simulink model "Final_EWASP_VC"  (R2022a)
settings: Solver=ode1  StartTime=0.0  StopTime=24*3600  FixedStep=10  RelTol=1e-3
values from neighbouring files (symbols this model uses):
  Aux_Threshold = 52    [Setup_Code_EWASP_VC.m]
  buildingAge = 2005    [Setup_Code_EWASP_VC.m]
  ceilingHeight = 2.4    [Setup_Code_EWASP_VC.m]
  conductiveHconnectMatrix = [ ... (first row only)    [Setup_Code_EWASP_VC.m]
  cRoofGreen = 100000    [Setup_Code_EWASP_VC.m]
  Defrost_After_Time = 30    [Setup_Code_EWASP_VC.m]
  DHWDemandProfile = occFreegainHotwaterElecTestPassiveOcc3(:,3)    [Setup_Code_EWASP_VC.m]
  Elec_Max = Elec_Max*(30/24.2)    [Setup_Code_EWASP_VC.m]
  Elec_Mid = Elec_Mid*(30/24.2)    [Setup_Code_EWASP_VC.m]
  Elec_Min = Elec_Min*(30/24.2)    [Setup_Code_EWASP_VC.m]
  ElecDemandProfile = occFreegainHotwaterElecTestPassiveOcc3(:,4)    [Setup_Code_EWASP_VC.m]
  ElecFixed = [Elec_Max(6,2) Elec_Max(6,4) Elec_Max(6,6) Elec_Max(6,7) ... (first row only)    [Setup_Code_EWASP_VC.m]
  floorOrCeilingArea = floorOrCeilingArea*1.15    [Setup_Code_EWASP_VC.m]
  forceCold = 0    [Setup_Code_EWASP_VC.m]
  freegain = occFreegainHotwaterElecTestPassiveOcc3(:,2)-max(occupancy)*25    [Setup_Code_EWASP_VC.m]
  furnitureModelOn = 1    [Setup_Code_EWASP_VC.m]
  Heat_Max = Heat_Max*(30/24.2)    [Setup_Code_EWASP_VC.m]
  Heat_Mid = Heat_Mid*(30/24.2)    [Setup_Code_EWASP_VC.m]
  Heat_Min = Heat_Min*(30/24.2)    [Setup_Code_EWASP_VC.m]
  HeatFixed = [Heat_Max(6,2) Heat_Max(6,4) Heat_Max(6,6) Heat_Max(6,7) ... (first row only)    [Setup_Code_EWASP_VC.m]
  HeatingOnProfile = repmat(HeatingOnProfile,365,1)    [Setup_Code_EWASP_VC.m]
  HEX_ReturnLowerLimit = 52.5    [Setup_Code_EWASP_VC.m]
  HEX_ReturnUpperLimit = 55    [Setup_Code_EWASP_VC.m]
  LeakMultiplier = 1+(2*(rand()-0.5)/10)    [Setup_Code_EWASP_VC.m]
  loopCap = 15    [Setup_Code_EWASP_VC.m]
  maxOcc = max(occupancyProfile)    [Setup_Code_EWASP_VC.m]
  NESW_wallArea = max(NESW_Lengths*ceilingHeight-NESW_Windows,0)    [Setup_Code_EWASP_VC.m]
  NESW_Windows = [ ... (first row only)    [Setup_Code_EWASP_VC.m]
  numRooms = roomCount    [Setup_Code_EWASP_VC.m]
  offsetDays = 0    [Setup_Code_EWASP_VC.m]
  pumpChoice = pumpChoices(MinIndex,1)    [Setup_Code_EWASP_VC.m]
  pumpRamp = 180    [Setup_Code_EWASP_VC.m]
  ReturnLowerLimit = 37.5    [Setup_Code_EWASP_VC.m]
  ReturnUpperLimit = 40    [Setup_Code_EWASP_VC.m]
  RoofIrradiance = Flat_NS_EW_RoofIrradiance(:,1)    [Setup_Code_EWASP_VC.m]
  roofStartTemp = ones(11,1)*20    [Setup_Code_EWASP_VC.m]
  rooftype = 0    [Setup_Code_EWASP_VC.m]
  RoomDataMatrix = [zeros(1,12);ones(1,12)*wallDensity;zeros(1,12);ones(1,12)*wallU;ones(1,12)*windowU;ones(1,12)*floorU;ones(1,12)*ceilingU;zeros(1,12);windowArea, 0;floorOrCeilingArea;zeros(1,12);floorOrCeilingArea*ceilingHeight]    [Setup_Code_EWASP_VC.m]
  roomVol = roomVol*1.15    [Setup_Code_EWASP_VC.m]
  slabStartTemp = (GroundTempTimeSeries(offsetDays*1440+1,1)+thermostatSetting)/2    [Setup_Code_EWASP_VC.m]
  SlackRequest = zeros(1440,1)    [Setup_Code_EWASP_VC.m]
  SolarThermalExists = 0    [Setup_Code_EWASP_VC.m]
  SourceFixed = HeatFixed-ElecFixed    [Setup_Code_EWASP_VC.m]
  StateSeries = StateSeriesGenerator(22,7,1)    [Setup_Code_EWASP_VC.m]
  Tank_Lower_Temp = 49.5    [Setup_Code_EWASP_VC.m]
  Tank_Upper_Temp = 52    [Setup_Code_EWASP_VC.m]
  Tank_Volume_m3 = 0.15    [Setup_Code_EWASP_VC.m]
  TankHeatHour = randi([1 5])-1    [Setup_Code_EWASP_VC.m]
  thermostatSetting = 20.0    (= 20)    [Setup_Code_EWASP_VC.m]
  upDown = [0;0;0;0;1;1;1;1;1;1;1]    [Setup_Code_EWASP_VC.m]
  variableASHP = 1    [Setup_Code_EWASP_VC.m]
  wallStartTempExt = thermostatSetting*(0.266+0.00215*outdoorStartTemp+0.018*wallU+0.00113*outdoorStartTemp*wallU+0.0068*wallU^2)    [Setup_Code_EWASP_VC.m]
undefined symbols (not defined in the file or in its folder): a, ceilingU, condUDMatrix, convUDMatrix, deltaPEXPANDED_E, deltaPEXPANDED_E2, deltaPEXPANDED_N, deltaPEXPANDED_N2, deltaPEXPANDED_S, deltaPEXPANDED_S2, deltaPEXPANDED_W, deltaPEXPANDED_W2, DesiredDHWTemp, DesiredFlowTempVsInOutDeltaTemp, DiffuseHorizontal, DiscIntNeverNeededParam, DNI, dwnAndConcrete, DWORK_A_HX, DWORK_CHK_FLU, DWORK_CP_NODE, DWORK_DH, DWORK_FLUID, DWORK_HCON, DWORK_LOSS, DWORK_MDOTDOWN, DWORK_MDOTIN, DWORK_MDOTUP, DWORK_MIX, DWORK_PRESS, DWORK_QDOTIN, DWORK_RHO_NODE, DWORK_TIN, DWORK_TS_OLD, DWORK_V_NODE, GroundTempTimeSeries, HCM, HCM2, HCM_closed, HCM_closed2, intermediateU, IsTop, massFlowMatrix, neighbourMatrix, numericalRoomUse, RadiatorMatrix, room2roomflowmatrix_E, room2roomflowmatrix_E2, room2roomflowmatrix_N, room2roomflowmatrix_N2, room2roomflowmatrix_S, room2roomflowmatrix_S2, room2roomflowmatrix_W, room2roomflowmatrix_W2, StateAirInEXPANDED_E, StateAirInEXPANDED_E2, StateAirInEXPANDED_N, StateAirInEXPANDED_N2, StateAirInEXPANDED_S, StateAirInEXPANDED_S2 ... (+23)
libraries: simulink x6, dspsigops x4, dspmtrx3 x4, carnot x3, spsEdgeDetectorLib x2, dspstat3 x2, powerlib_meascontrol x1, simulink_extras x1
(part 1 of 27)
settings Model: Creator=cpp14rcj  LastModifiedBy=cpp14rcj
settings SolverCC: AlgebraicLoopSolver=TrustRegion  AutoInsertRateTranBlk=on
settings DataIOCC: SaveFormat=Array  ReturnWorkspaceOutputs=off
settings OptimizationCC: DefaultParameterBehavior=Inlined
settings DebuggingCC: UnconnectedInputMsg=warning  UnconnectedOutputMsg=warning  UnconnectedLineMsg=warning  SFMachineParentedDataDiag=warning  ArithmeticOperatorsInVariantConditions=warning
settings SFSimCC: CustomCodeUndefinedFunction=UseInterfaceOnly
settings ConfigComp: PSAutoStubLUT=on

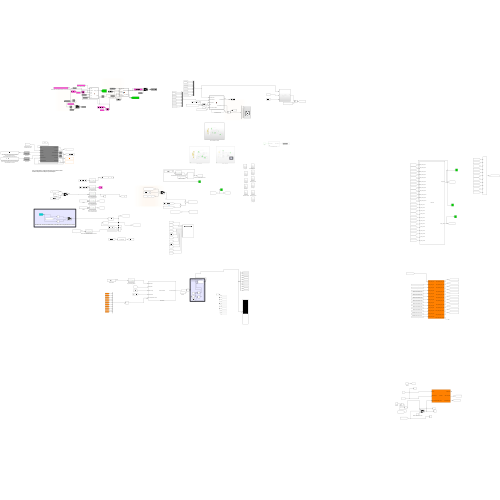
[thumbnail: Simulink's stored preview of the top-level diagram]
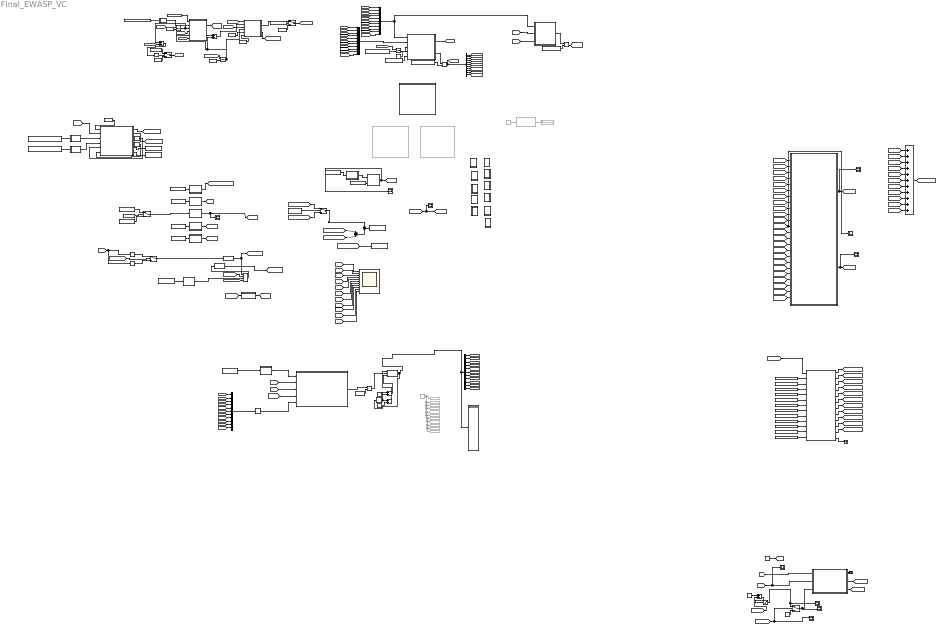
== system Final_EWASP_VC ==
  note: Prevents airflow from altering
      | extremely rapidly
  note: Handles the room thermostat band, and relaxes it if a request to do so is sent
  note: Grey Components: Components that are part of the model
      | White Components: Example Inputs/Outputs
  1 m : Relay  OnSwitchValue=18.1  OffSwitchValue=18  OnOutputValue=0  OffOutputValue=1  OutDataTypeStr=boolean
  1 m10 : Relay  OnSwitchValue=7  OffSwitchValue=1  OutDataTypeStr=boolean
  ASHP_Subsystem : Subsystem  Commented=on
  ASHP_Subsystem_Variable : Subsystem
  Add : Sum  Inputs=11
  Add2 : Sum
  Add3 : Sum  Inputs=+-
  Airflow Model : Subsystem
      mask Display:
      | disp('Air Flow Heat Loss')
      | port_label('input',1,'State Switch')
      | port_label('input',2,'Wind Speed')
      | port_label('input',3,'Outdoor Temp')
      | port_label('input',4,'Wind Direction')
      | port_label('input',5,'Room Temperature Vector')
      | port_label('output',1,'Room Loss Vector')
  CondLossIntermediate : Subsystem  Commented=on
      mask Display:
      | port_label('input',1, 'RoomNum')
      | port_label('output',1,'IntCondGain')
  Constant1 : Constant  Commented=on  Value=0
  Constant10 : Constant  Value=50
  Constant11 : Constant  Value=maxOcc*0.054/2
  Constant12 : Constant  Value=variableASHP
  Constant14 : Constant  Value=0
  Constant2 : Constant  Value=25
  Constant3 : Constant  Value=2.1
  Constant4 : Constant  Commented=on  Value=11
  Constant5 : Constant  Value=25
  Constant6 : Constant  Value=20*ones(11,11)
  Constant7 : Constant  Value=conductiveHconnectMatrix
  Constant8 : Constant  Value=0
  Constant9 : Constant  Value=20
  Data Type Conversion : DataTypeConversion  OutDataTypeStr=double  SaturateOnIntegerOverflow=off  RndMeth=Floor
  Data Type Conversion2 : DataTypeConversion  OutDataTypeStr=double  SaturateOnIntegerOverflow=off  RndMeth=Floor
  Delay3 : Delay  DelayLength=1  InitialCondition=0
  Delay4 : Delay  DelayLength=1  InitialCondition=0
  Delay5 : Delay  DelayLength=1  InitialCondition=0
  Demux : Demux  Outputs=11
  Demux1 : Demux  Outputs=11
  Digital Clock3 : DigitalClock  SampleTime=10
  Discrete-Time Integrator : DiscreteIntegrator  InitialConditionSource=external  InitialCondition=20  SampleTime=-1  ICPrevOutput=DiscIntNeverNeededParam  ICPrevScaledInput=DiscIntNeverNeededParam
  Discrete-Time Integrator1 : DiscreteIntegrator  InitialConditionSource=external  SampleTime=-1  ICPrevOutput=DiscIntNeverNeededParam  ICPrevScaledInput=DiscIntNeverNeededParam
  Display : Display
  Display3 : Display  Commented=on
  GSHP_Subsystem : Subsystem  Commented=on
  Goto11 : Goto  Commented=on  GotoTag=AirLoss5  TagVisibility=global
  Goto12 : Goto  Commented=on  GotoTag=AirLoss6  TagVisibility=global
  Goto16 : Goto  Commented=on  GotoTag=AirLoss7  TagVisibility=global
  Goto18 : Goto  Commented=on  GotoTag=AirLoss8  TagVisibility=global
  Goto19 : Goto  Commented=on  GotoTag=AirLoss9  TagVisibility=global
  Goto20 : Goto  Commented=on  GotoTag=AirLoss10  TagVisibility=global
  Goto21 : Goto  Commented=on  GotoTag=AirLoss11  TagVisibility=global
  Goto5 : Goto  Commented=on  GotoTag=AirLoss1  TagVisibility=global
  Goto7 : Goto  Commented=on  GotoTag=AirLoss2  TagVisibility=global
  Goto8 : Goto  Commented=on  GotoTag=AirLoss3  TagVisibility=global
  Goto9 : Goto  Commented=on  GotoTag=AirLoss4  TagVisibility=global
  Heat sys act?1 : Constant  Value=HeatingOnProfile
  Heat sys act?2 : Constant  Value=StateSeries
  Logical Operator5 : Logic  Inputs=4  AllPortsSameDT=off  OutDataTypeStr=boolean
  MATLAB Function : MATLAB Function  TreatAsAtomicUnit=on
  MATLAB Function1 : MATLAB Function  TreatAsAtomicUnit=on
  MATLAB Function2 : MATLAB Function  TreatAsAtomicUnit=on
  MATLAB Function3 : MATLAB Function  TreatAsAtomicUnit=on
  Massflow when system is off3 : Constant  Value=0
  Massflow when system is on1 : Constant  Value=massFlowMatrix(1,3)
  Massflow when system is on10 : Constant  Value=massFlowMatrix(1,11)
  Massflow when system is on11 : Constant  Value=massFlowMatrix(1,10)
  Massflow when system is on13 : Constant  Value=massFlowMatrix(1,2)
  Massflow when system is on2 : Constant  Value=massFlowMatrix(1,1)
  Massflow when system is on3 : Constant  Value=massFlowMatrix(1,6)
  Massflow when system is on4 : Constant  Value=massFlowMatrix(1,5)
  Massflow when system is on5 : Constant  Value=massFlowMatrix(1,9)
  Massflow when system is on6 : Constant  Value=massFlowMatrix(1,8)
  Massflow when system is on7 : Constant  Value=massFlowMatrix(1,4)
  Massflow when system is on8 : Constant  Value=massFlowMatrix(1,7)
  Massflow when system is on9 : Constant  Value=massFlowMatrix(1,12)
  Minus : Sum  Inputs=+-
  Mux : Mux  Inputs=11
  Mux1 : Mux  Inputs=11
  Offset Independent time series element selector : Subsystem
  Offset Independent time series element selector1 : Subsystem
  Offset Independent time series element selector2 : Subsystem
  Plus : Sum  Inputs=+-
  Plus1 : Sum  Inputs=+-
  Product : Product  Inputs=*/
  Product2 : Product
  Product3 : Product  Inputs=*/
  Product4 : Product  Inputs=*/
  Radiator w/Thermostatic Control : Subsystem  mask{DeltaT_Nominal=40, Power_Nominal=100, TRV_Therm_Setpoint=1000, Water_Volume=10}
      mask prompts: DeltaT_Nominal "DeltaT_Nominal (oC)"; Power_Nominal "Power_Nominal (W)"; TRV_Therm_Setpoint "TRV/Thermostat Setpoint (oC)"; Water_Volume "Water Volume (l)"
      mask Display:
      | disp('Radiator')
      | port_label('input', 1, 'Troom')
      | port_label('input', 2, 'Water Temp In')
      | port_label('input', 3, 'Water Mass Flow Rate (open)')
      | port_label('output', 1, 'Qdot2room')
      | port_label('output', 2, 'Water Temp Out')
      | port_label('output', 3, 'Actual Mass Flow')
      | %image('C:\Users\cpp14rcj\Desktop\MODEL IMAGES\radiator-67-778961.png')
  Relay1 : Relay  OnSwitchValue=thermostatSetting  OffSwitchValue=thermostatSetting-thermostatBand  OnOutputValue=0  OffOutputValue=1  OutDataTypeStr=boolean
  Saturation Dynamic : simulink/Discontinuities/Saturation Dynamic  OutMin=[]  OutMax=[]  OutDataTypeStr=Inherit: Same as second input  OutDataType=fixdt(1, 16)  OutScaling=2^-10  DoSatur=off
  Saturation1 : Saturate  UpperLimit=1000  LowerLimit=0
  Scope{,3,6,10,12..13,16,19} (8 alike) : Scope
  Scope5 : Scope  NumInputPorts=11
  Scope7 : Scope  NumInputPorts=2
  Scope9 : Scope  NumInputPorts=2
  Select Correct Element from Array1 : Subsystem
  Select Correct Element from Array2 : Subsystem
  "Select correct element from array, considering offset" : Subsystem
  "Select correct element from array, considering offset1" : Subsystem
  "Select correct element from array, considering offset2" : Subsystem
  "Select correct element from array, considering offset3" : Subsystem
  "Select correct element from array, considering offset4" : Subsystem
  Selector2 : Selector  NumberOfDimensions=2  InputPortWidth=3  IndexOptions=Index vector (dialog),Index vector (dialog)  Indices=1:11,1  OutputSizes=1,1
  Subsystem : Subsystem
      mask Display:
      | disp('Flow mixer')
      | port_label('input', 13, 'T_return_rad1')
      | port_label('input', 14, 'T_return_rad2')
      | port_label('input', 15, 'T_return_rad3')
      | port_label('input', 16, 'T_return_rad4')
      | port_label('input', 17, 'T_return_rad5')
      | port_label('input', 18, 'T_return_rad6')
      | port_label('input', 19, 'T_return_rad7')
      | port_label('input', 20, 'T_return_rad8')
      | port_label('input', 21, 'T_return_rad9')
      | port_label('input', 22,'T_return_rad10')
      | port_label('input', 23,'T_return_rad11')
      | port_label('input', 24,'T_return_rad12')
      | 
      | port_label('input', 1, 'mdot_return_rad1')
      | port_label('input', 2, 'mdot_return_rad2')
      | port_label('input', 3, 'mdot_return_rad3')
      | port_label('input', 4, 'mdot_return_rad4')
      | port_label('input', 5, 'mdot_return_rad5')
      | port_label('input', 6, 'mdot_return_rad6')
      | port_label('input', 7, 'mdot_return_rad7')
      | port_label('input', 8, 'mdot_return_rad8')
      | port_label('input', 9, 'mdot_return_rad9')
      | port_label('input', 10, 'mdot_return_rad10')
      | port_label('input', 11, 'mdot_return_rad11')
      | port_label('input', 12, 'mdot_return_rad12')
      | 
      | port_label('output', 1, 'mdot_total')
      | port_label('output', 2, 'Temp_mixed')
  Subsystem1 : Subsystem
      mask Display:
      | port_label('input', 1, 'mdot_return_rad1')
      | port_label('input', 2, 'mdot_open_rad1')
      | port_label('input', 3, 'mdot_open_rad2')
      | port_label('input', 4, 'mdot_open_rad3')
      | port_label('input', 5, 'mdot_open_rad4')
      | port_label('input', 6, 'mdot_open_rad5')
      | port_label('input', 7, 'mdot_open_rad6')
      | port_label('input', 8, 'mdot_open_rad7')
      | port_label('input', 9, 'mdot_open_rad8')
      | port_label('input', 10, 'mdot_open_rad9')
      | port_label('input', 11, 'mdot_open_rad10')
      | port_label('input', 12, 'mdot_open_rad11')
      | port_label('input', 13, 'mdot_open_rad12')
      | 
      | 
      | port_label('output', 1, 'mdot_actual_open_rad1')
      | port_label('output', 2, 'mdot_actual_open_rad2')
      | port_label('output', 3, 'mdot_actual_open_rad3')
      | port_label('output', 4, 'mdot_actual_open_rad4')
      | port_label('output', 5, 'mdot_actual_open_rad5')
      | port_label('output', 6, 'mdot_actual_open_rad6')
      | port_label('output', 7, 'mdot_actual_open_rad7')
      | port_label('output', 8, 'mdot_actual_open_rad8')
      | port_label('output', 9, 'mdot_actual_open_rad9')
      | port_label('output', 10, 'mdot_actual_open_rad10')
      | port_label('output', 11, 'mdot_actual_open_rad11')
      | port_label('output', 12, 'mdot_actual_open_rad12')
  Subsystem2 : Subsystem
      mask Display: disp('10 min Limiter')
  Subsystem3 : Subsystem
  Subsystem4 : Subsystem
  Subsystem_Room1 : Subsystem
  Subsystem_Room10 : Subsystem
  Subsystem_Room11 : Subsystem
  Subsystem_Room2 : Subsystem
  Subsystem_Room3 : Subsystem
  Subsystem_Room4 : Subsystem
  Subsystem_Room5 : Subsystem
  Subsystem_Room6 : Subsystem
  Subsystem_Room7 : Subsystem
  Subsystem_Room8 : Subsystem
  Subsystem_Room9 : Subsystem
  Sum1 : Sum
  Sum2 : Sum
  Switch{,1..4,7} (6 alike) : Switch  Criteria=u2 > Threshold  Threshold=0.5  SaturateOnIntegerOverflow=off  InputSameDT=off
  Temp Hex : DiscreteIntegrator  InitialConditionSource=external  InitialCondition=20  SampleTime=-1  ICPrevOutput=DiscIntNeverNeededParam  ICPrevScaledInput=DiscIntNeverNeededParam
  Terminator1 : Terminator
  Terminator13 : Terminator
  Tinitial10 : Constant  Value=0.2
  Tinitial16 : Constant  Value=20
  Tinitial18 : Constant  Value=LeakMultiplier
  To Workspace3 : ToWorkspace  VariableName=MO1  SaveFormat=Timeseries  SampleTime=-1
  To Workspace4 : ToWorkspace  VariableName=MO2  SaveFormat=Timeseries  SampleTime=-1
  To Workspace7 : ToWorkspace  VariableName=HP_Elec  SaveFormat=Timeseries  SampleTime=-1
  To Workspace8 : ToWorkspace  VariableName=Other_Elec  SaveFormat=Timeseries  SampleTime=-1
  Vector Concatenate : Concatenate  NumInputs=11
  angle that DNI hits a NEWS wall/window as a function of time1 : Constant  Value=RoofIrradiance
  angle that DNI hits a NEWS wall/window as a function of time2 : Constant  Value=SolarThermalExists
  assign 1m2 per occupant : Constant  Value=maxOcc
  coil watermass - roughly 8m coil with 9mm diameter : Constant  Value=0.55
  effective coil HEX u value : Constant  Value=11
  on? (I/O)1 : Constant  Value=GroundTempTimeSeries  OutDataTypeStr=double
  on? (I/O)2 : Constant  Value=5*ones(525600,1)  OutDataTypeStr=double
  on? (I/O)3 : Constant  Value=windSpeedSeries  OutDataTypeStr=double
  on? (I/O)4 : Constant  Value=WDS_Numerical  OutDataTypeStr=double
  on? (I/O)5 : Constant  Value=ElecDemandProfile  OutDataTypeStr=double
  on? (I/O)6 : Constant  Value=TemperatureSeries  OutDataTypeStr=double
  on? (I/O)7 : Constant  Value=forceCold  OutDataTypeStr=double
  roomAirHeatCapcities : Constant  Value=1000*1.225*roomVol(1,1:11)'
  roomAirHeatCapcities1 : Constant  Value=1000*1.225*roomVol(1,1:11)'
  "vector Representing request to charge a 2kWh (7.2 MJ) (vector results in charging between 00:00 and 03:00, and brings battery to 75% SoC" : Constant  Value=[zeros(1440,1)]
  vector Representing request to slacken deadband at any given minute of the day (sends request between 18:00 and 21:00) : Constant  Value=SlackRequest
  watts per occupant : Constant  Value=freegain  OutDataTypeStr=double
  watts per occupant1 : Constant  Value=numRooms  OutDataTypeStr=double
  tag scope: AirLoss10=global, AirLoss11=global, AirLoss1=global, AirLoss2=global, AirLoss3=global, AirLoss4=global, AirLoss5=global, AirLoss6=global, AirLoss7=global, AirLoss8=global, AirLoss9=global, Allowed_on=global, Global_Control_Signal=global, Ground=global, MassFlowTotal=global, MassFlow_Full_Open_10=global, MassFlow_Full_Open_11=global, MassFlow_Full_Open_1=global, MassFlow_Full_Open_2=global, MassFlow_Full_Open_3=global, MassFlow_Full_Open_4=global, MassFlow_Full_Open_5=global, MassFlow_Full_Open_6=global, MassFlow_Full_Open_7=global, MassFlow_Full_Open_8=global, MassFlow_Full_Open_9=global, Mdot_Actual_12=global, MixedTemp=global, Occ_Free_Gain=global, RAD_TOTAL=global, SolarHeatToWater=global, THB_In=global, T_12=global, T_Out=global, T_return_R12=global, deltaTPartition10=global, deltaTPartition11=global, deltaTPartition1=global, deltaTPartition2=global, deltaTPartition3=global, deltaTPartition4=global, deltaTPartition5=global, deltaTPartition6=global, deltaTPartition7=global, deltaTPartition8=global, deltaTPartition9=global, deltaTRoofNodes=global, pump_control_signal=global, windDirection=global, windSpeed=global
  wires:
  Data Type Conversion2/1 -> [pump_control_signal], Logical Operator5/1
  Logical Operator5/1 -> Data Type Conversion/1
  [Allowed_on] -> Logical Operator5/2
  Subsystem/2(Out2) -> Scope12/1, [MixedTemp]
  [T_return_R12] -> Subsystem/24(In24)
  [T_return_R11] -> Subsystem/23(In23)
  [T_return_R6] -> Subsystem/18(In18)
  [T_return_R7] -> Subsystem/19(In19)
  [T_return_R8] -> Subsystem/20(In20)
  [T_return_R9] -> Subsystem/21(In21)
  [T_return_R4] -> Subsystem/16(In16)
  [T_return_R1] -> Subsystem/13(In13)
  [Mdot_Actual_11] -> Subsystem/11(In11)
  [Mdot_Actual_12] -> Scope19/1, Subsystem/12(In12)
  [Mdot_Actual_8] -> Subsystem/8(In8)
  [T_return_R5] -> Subsystem/17(In17)
  [Mdot_Actual_5] -> Subsystem/5(In5)
  [Mdot_Actual_6] -> Subsystem/6(In6)
  [Mdot_Actual_4] -> Subsystem/4(In4)
  [Mdot_Actual_10] -> Subsystem/10(In10)
  [Mdot_Actual_3] -> Subsystem/3(In3)
  [Mdot_Actual_2] -> Subsystem/2(In2)
  [T_return_R10] -> Subsystem/22(In22)
  [Mdot_Actual_9] -> Subsystem/9(In9)
  [Mdot_Actual_1] -> Subsystem/1(In1)
  [T_return_R3] -> Subsystem/15(In15)
  [Mdot_Actual_7] -> Subsystem/7(In7)
  [T_return_R2] -> Subsystem/14(In14)
  [THB_In_Pre] -> [THB_In], Scope16/1
  [pump_control_signal] -> Subsystem1/1(In1)
  Massflow when system is on2/1 -> Subsystem1/2(In2)
  Massflow when system is on13/1 -> Subsystem1/3(In3)
  Massflow when system is on1/1 -> Subsystem1/4(In4)
  Subsystem1/1(Out1) -> [MassFlow_Full_Open_1]
  Subsystem1/2(Out2) -> [MassFlow_Full_Open_2]
  Subsystem1/3(Out3) -> [MassFlow_Full_Open_3]
  Subsystem1/4(Out4) -> [MassFlow_Full_Open_4]
  Subsystem1/5(Out5) -> [MassFlow_Full_Open_5]
  Subsystem1/6(Out6) -> [MassFlow_Full_Open_6]
  Subsystem1/7(Out7) -> [MassFlow_Full_Open_7]
  Subsystem1/8(Out8) -> [MassFlow_Full_Open_8]
  Subsystem1/9(Out9) -> [MassFlow_Full_Open_9]
  Subsystem1/11(Out11) -> [MassFlow_Full_Open_11]
  Subsystem1/12(Out12) -> Terminator13/1
  Data Type Conversion/1 -> [Global_Control_Signal]
  Subsystem/1(Out1) -> Scope10/1, [MassFlowTotal]
  [T_4] -> Scope5/4
  [T_5] -> Scope5/5
  [T_6] -> Scope5/6
  [T_1] -> Scope5/1
  [T_2] -> Scope5/2
  [T_3] -> Scope5/3
  [T_7] -> Scope5/7
  [T_8] -> Scope5/8
  [T_9] -> Scope5/9
  [T_10] -> Scope5/10
  [T_11] -> Scope5/11
  [hysteresis] -> Subsystem2/1(In1)
  Subsystem2/1(Out1) -> [Allowed_on]
  Tinitial16/1 -> [T_12]
  [T_12] -> Radiator w/Thermostatic Control/1(In1)
  [THB_In] -> Scope/1, Radiator w/Thermostatic Control/2(In2)
  Tinitial10/1 -> Minus/1
  Minus/1 -> Saturation1/1
  [RAD_TOTAL] -> Minus/2
  Saturation1/1 -> Scope3/1, Switch7/1
  Radiator w/Thermostatic Control/2(Out2) -> [T_return_R12]
  Radiator w/Thermostatic Control/3(Out3) -> [Mdot_Actual_12]
  Subsystem1/10(Out10) -> [MassFlow_Full_Open_10]
  Add/1 -> [RAD_TOTAL]
  Massflow when system is off3/1 -> Switch7/3
  [pump_control_signal] -> Scope9/1, Switch7/2
  Switch7/1 -> Scope7/2, Radiator w/Thermostatic Control/3(In3)
  [Mdot_Actual_2] -> Add/2
  [Mdot_Actual_4] -> Add/4
  [Mdot_Actual_7] -> Add/7
  [Mdot_Actual_9] -> Add/9
  [Mdot_Actual_11] -> Add/11
  [Mdot_Actual_6] -> Add/6
  [Mdot_Actual_8] -> Add/8
  [Mdot_Actual_10] -> Add/10
  [Mdot_Actual_1] -> Add/1
  [Mdot_Actual_3] -> Add/3
  [Mdot_Actual_5] -> Add/5
  Constant4/1 -> CondLossIntermediate/1(In1)
  CondLossIntermediate/1(Out1) -> Display3/1
  [windDirection] -> Airflow Model/4(In4)
  Vector Concatenate/1 -> Selector2/1
  Heat sys act?2/1 -> "Select correct element from array, considering offset4"/1(In1)
  [T_Out] -> Airflow Model/3(In3)
  Demux/1 -> [AirLoss1]
  Demux/2 -> [AirLoss2]
  Demux/3 -> [AirLoss3]
  Demux/4 -> [AirLoss4]
  Demux/5 -> [AirLoss5]
  Demux/6 -> [AirLoss6]
  Demux/7 -> [AirLoss7]
  Demux/8 -> [AirLoss8]
  Demux/9 -> [AirLoss9]
  Demux/10 -> [AirLoss10]
  Demux/11 -> [AirLoss11]
  [T_1] -> Vector Concatenate/1
  [T_2] -> Vector Concatenate/2
  [T_3] -> Vector Concatenate/3
  [T_4] -> Vector Concatenate/4
  [T_5] -> Vector Concatenate/5
  [T_6] -> Vector Concatenate/6
  [T_7] -> Vector Concatenate/7
  [T_8] -> Vector Concatenate/8
  [T_9] -> Vector Concatenate/9
  [T_10] -> Vector Concatenate/10
  [T_11] -> Vector Concatenate/11
  Selector2/1 -> Airflow Model/5(In5)
  "Select correct element from array, considering offset4"/1(Out1) -> Airflow Model/1(In1)
  on? (I/O)1/1 -> "Select correct element from array, considering offset"/1(In1)
  on? (I/O)3/1 -> "Select correct element from array, considering offset2"/1(In1)
  "Select correct element from array, considering offset3"/1(Out1) -> [windDirection]
  on? (I/O)4/1 -> "Select correct element from array, considering offset3"/1(In1)
  "Select correct element from array, considering offset"/1(Out1) -> [Ground]
  [windSpeed] -> Airflow Model/2(In2)
  Radiator w/Thermostatic Control/1(Out1) -> Terminator1/1
  on? (I/O)5/1 -> Offset Independent time series element selector/1(In1)
  Offset Independent time series element selector/1(Out1) -> [ApplianceAndLightElectricalPower]
  Offset Independent time series element selector1/1(Out1) -> Logical Operator5/3
  Heat sys act?1/1 -> Offset Independent time series element selector1/1(In1)
  Product2/1 -> Saturation Dynamic/2
  Tinitial18/1 -> Product2/2
  [ElectrifiedHeatToWater] -> Sum2/1
  Airflow Model/1(Out1) -> Product2/1
  Massflow when system is on3/1 -> Subsystem1/7(In7)
  Massflow when system is on4/1 -> Subsystem1/6(In6)
  Massflow when system is on7/1 -> Subsystem1/5(In5)
  Massflow when system is on11/1 -> Subsystem1/11(In11)
  Massflow when system is on9/1 -> Subsystem1/13(In13)
  Massflow when system is on10/1 -> Subsystem1/12(In12)
  Massflow when system is on5/1 -> Subsystem1/10(In10)
  Massflow when system is on6/1 -> Subsystem1/9(In9)
  Massflow when system is on8/1 -> Subsystem1/8(In8)
  [AuxHeatToWater] -> Sum2/2
  Delay4/1 -> MATLAB Function/6(ModelFeedbackIn2)
  Digital Clock3/1 -> MATLAB Function/1(clock)
  vector Representing request to slacken deadband at any given minute of the day (sends request between 18:00 and 21:00)/1 -> Select Correct Element from Array1/1(In1)
  "vector Representing request to charge a 2kWh (7.2 MJ) (vector results in charging between 00:00 and 03:00, and brings battery to 75% SoC"/1 -> Select Correct Element from Array2/1(In1)
  Delay3/1 -> MATLAB Function/5(ModelFeedbackIn)
  MATLAB Function/4(ModelFeedbackOut2) -> Delay4/1
  MATLAB Function/6(MonitorOut2) -> To Workspace4/1
  MATLAB Function/2(RelaxBand) -> [RelaxBand]
  Select Correct Element from Array2/1(Out1) -> MATLAB Function/4(ExternalIn2)
  Select Correct Element from Array1/1(Out1) -> MATLAB Function/3(ExternalIn)
  MATLAB Function/5(MonitorOut) -> To Workspace3/1
  MATLAB Function/3(ModelFeedbackOut) -> Delay3/1
  [T_5] -> MATLAB Function/2(HeatSysIn)
  [SystemActiveInterractor] -> Logical Operator5/4
  Switch/1 -> Data Type Conversion2/1
  Relay1/1 -> Switch/3
  [T_6] -> Relay1/1, 1 m/1
  1 m/1 -> Switch/1
  [RelaxBand] -> Switch/2
  Constant1/1 -> Goto21/1, Goto20/1, Goto19/1, Goto18/1, Goto16/1, Goto12/1, Goto11/1, Goto9/1, Goto8/1, Goto7/1, Goto5/1
  Delay5/1 -> Add3/1, Add2/1
  Constant2/1 -> Add3/2
  Constant5/1 -> Add2/2
  Add3/1 -> Saturation Dynamic/3
  Add2/1 -> Saturation Dynamic/1
  "Select correct element from array, considering offset1"/1(Out1) -> Scope13/1, [T_Out]
  MATLAB Function/1(SystemActive) -> [SystemActiveInterractor]
  Switch4/1 -> Sum1/1
  watts per occupant1/1 -> Product/2
  Product/1 -> Scope6/1, [Occ_Free_Gain]
  watts per occupant/1 -> Offset Independent time series element selector2/1(In1)
  Offset Independent time series element selector2/1(Out1) -> Product/1
  [ApplianceAndLightElectricalPower] -> To Workspace8/1
  Saturation Dynamic/1 -> Delay5/1, Display/1, Demux/1
  "Select correct element from array, considering offset2"/1(Out1) -> [windSpeed]
  [Q_rad_win11] -> Mux1/11
  [Q_rad_win2] -> Mux1/2
  [Q_rad_win5] -> Mux1/5
  [Q_rad_win8] -> Mux1/8
  [Q_rad_win3] -> Mux1/3
  Demux1/3 -> [deltaTPartition3]
  Demux1/11 -> [deltaTPartition11]
  Demux1/9 -> [deltaTPartition9]
  [Q_rad_win6] -> Mux1/6
  Demux1/6 -> [deltaTPartition6]
  Demux1/5 -> [deltaTPartition5]
  Demux1/8 -> [deltaTPartition8]
  Discrete-Time Integrator1/1 -> MATLAB Function1/3(wallTempOuter)
  Mux1/1 -> MATLAB Function1/2(irradianceToRoom)
  Demux1/7 -> [deltaTPartition7]
  [T_8] -> Mux/8
  [T_3] -> Mux/3
  [T_2] -> Mux/2
  MATLAB Function1/2(RoomHeatLossVector) -> Product3/1
  Demux1/4 -> [deltaTPartition4]
  [T_10] -> Mux/10
  Demux1/1 -> [deltaTPartition1]
  [T_6] -> Mux/6
  roomAirHeatCapcities/1 -> Product3/2
  Demux1/10 -> [deltaTPartition10]
  [deltaTWalls] -> Discrete-Time Integrator1/1
  Product3/1 -> [deltaTRoom], Demux1/1
  Constant7/1 -> MATLAB Function1/5(conductiveHconnectMatrix)
  [T_5] -> Mux/5
  [T_11] -> Mux/11
  [T_4] -> Mux/4
  [Q_rad_win9] -> Mux1/9
  [T_9] -> Mux/9
  [Q_rad_win1] -> Mux1/1
  [T_7] -> Mux/7
  [Q_rad_win4] -> Mux1/4
  [Q_rad_win7] -> Mux1/7
  Constant3/1 -> MATLAB Function1/4(wallU)
  [Q_rad_win10] -> Mux1/10
  Demux1/2 -> [deltaTPartition2]
  [T_1] -> Mux/1
  Constant6/1 -> Discrete-Time Integrator1/2
  MATLAB Function1/1(SurfaceDeltaT) -> [deltaTWalls]
  Mux/1 -> Subsystem3/1(In1), MATLAB Function1/1(RoomTempVector)
  [T_Out] -> Subsystem3/3(In3)
  [windSpeed] -> Subsystem3/2(In2)
  Subsystem3/1(Out1) -> Product4/1
  roomAirHeatCapcities1/1 -> Product4/2
  Product4/1 -> [deltaTRoofNodes]
  angle that DNI hits a NEWS wall/window as a function of time2/1 -> Switch3/2
  [tank_bottom_temp] -> MATLAB Function3/1(T_bottom_Tank)
  Subsystem4/1(Out1) -> MATLAB Function2/2(Q_SOLAR)
  Constant8/1 -> Switch3/3
  Switch3/1 -> [SolarHeatToWater]
  angle that DNI hits a NEWS wall/window as a function of time1/1 -> Subsystem4/1(In1)
  Constant10/1 -> Temp Hex/2
  effective coil HEX u value/1 -> MATLAB Function3/5(Hex_Uval)
  [T_Out] -> MATLAB Function2/4(T_amb)
  [dT_HEXsolar] -> Temp Hex/1
  Constant9/1 -> Discrete-Time Integrator/2
  Temp Hex/1 -> MATLAB Function3/4(Hex_Temp), MATLAB Function2/5(T_inlet), Plus/2
  MATLAB Function3/1(solarHeatToWater) -> Switch3/1
  Switch2/1 -> [mDotPanel]
  Discrete-Time Integrator/1 -> MATLAB Function2/3(T_panel), Plus1/1
  Constant14/1 -> Switch2/3
  Plus1/1 -> 1 m10/1
  assign 1m2 per occupant/1 -> MATLAB Function2/1(A_COLL)
  MATLAB Function2/1(delta_T_Panel) -> [dT_Panel]
  Plus/1 -> MATLAB Function3/2(T_diff)
  1 m10/1 -> Switch2/2
  [tank_bottom_temp] -> Plus1/2
  [mDotPanel] -> MATLAB Function2/6(m_dot)
  coil watermass - roughly 8m coil with 9mm diameter/1 -> MATLAB Function3/6(coilWaterMass)
  [mDotPanel] -> MATLAB Function3/3(mDotPanel)
  [dT_Panel] -> Discrete-Time Integrator/1
  MATLAB Function3/2(dT_HEXsolar) -> [dT_HEXsolar]
  Constant11/1 -> Switch2/1
  MATLAB Function2/2(T_outlet) -> Plus/1
  on? (I/O)2/1 -> Switch1/1
  Sum1/1 -> To Workspace7/1
  Sum2/1 -> Sum1/2
  on? (I/O)6/1 -> Switch1/3
  on? (I/O)7/1 -> Switch1/2
  Switch1/1 -> "Select correct element from array, considering offset1"/1(In1)
  [ElectrifiedHeatToSpace] -> Switch4/3
  [ElectrifiedHeatToSpaceV] -> Switch4/1
  Constant12/1 -> Switch4/2

== system Final_EWASP_VC/ASHP_Subsystem ==
  DHW for ASHP Case : Subsystem
  Defrost Timer : Subsystem
  Delay : Delay  DelayLength=1  InitialCondition=0
  Delay1 : Delay  DelayLength=1  InitialCondition=0
  Delay2 : Delay  DelayLength=5  InitialCondition=0
  Discrete-Time Integrator : DiscreteIntegrator  ExternalReset=falling  SampleTime=-1  LimitOutput=on  UpperSaturationLimit=1  LowerSaturationLimit=0  ICPrevOutput=DiscIntNeverNeededParam  ICPrevScaledInput=DiscIntNeverNeededParam
  Divide : Product  Inputs=*/
  Heat sys act? : Constant
  Logical Operator : Logic  Operator=NOT  Inputs=1  AllPortsSameDT=off  OutDataTypeStr=boolean
  Saturation : Saturate  UpperLimit=1  LowerLimit=0
  Scope2 : Scope
  Subsystem14 : Subsystem  TreatAsAtomicUnit=on
      mask Display:
      | port_label('input', 1, 'T_Out')
      | port_label('input', 2, 'NormalOn')
      | port_label('input', 3, 'DefrostOn')
      | port_label('input', 4, 'MixedTemp')
      | port_label('input', 5, 'MassFlowTotal')
      | port_label('input', 6, 'GCS')
      | port_label('input', 7, 'SHSig')
      | 
      | 
      | port_label('output', 1, 'Hysteresis')
      | port_label('output', 2, 'THB_to_Pre')
      | port_label('output', 3, 'd_signal')
      | port_label('output', 4, 'n_signal')
      | port_label('output', 5, 'Therm_out')
      | port_label('output', 6, 'Elec_out')
      | 
      | disp('SH_ASHP')
  Sum1 : Sum
  Sum2 : Sum  Inputs=2
  Sum3 : Sum
  Sum4 : Sum
  Time in seconds for Heat pump to reach full stady state output : Constant  Value=pumpRamp
  Water Demand Time Series (Minute) : Constant  Value=DHWDemandProfile
  mains water temp : Constant  Value=12
  tag scope: AuxHeatToWater=global, DHW_heating_on=global, DefrostOn=global, ElectrifiedHeatToSpace=global, HeatToSpace=global, HeatToWater=global, NormalOn=global, SH_Signal=global, THB_In_Pre=global, d_signal=global, hysteresis=global, n_signal=global, pump_power_Fraction=global
  wires:
  [n_signal] -> Delay1/1
  Time in seconds for Heat pump to reach full stady state output/1 -> Divide/2
  Subsystem14/1(Out1) -> [hysteresis]
  Sum1/1 -> Sum4/1, [d_signal]
  Saturation/1 -> Defrost Timer/3(In3)
  [d_signal] -> Delay/1
  Sum4/1 -> Discrete-Time Integrator/2, Divide/1
  [T_Out] -> Subsystem14/1(In1)
  Subsystem14/5(Out5) -> [HeatToSpace]
  Discrete-Time Integrator/1 -> Delay2/1
  [SH_Signal] -> Subsystem14/7(In7)
  [T_Out] -> DHW for ASHP Case/2(In2)
  DHW for ASHP Case/6(Out6) -> [AuxHeatToWater]
  Delay2/1 -> [pump_power_Fraction]
  Subsystem14/2(Out2) -> [THB_In_Pre]
  [MixedTemp] -> Subsystem14/4(In4)
  [pump_power_Fraction] -> Subsystem14/8(In8)
  Subsystem14/4(Out4) -> Sum3/1
  Water Demand Time Series (Minute)/1 -> DHW for ASHP Case/5(In5)
  [Global_Control_Signal] -> Subsystem14/6(In6)
  Divide/1 -> Discrete-Time Integrator/1
  Subsystem14/6(Out6) -> [ElectrifiedHeatToSpace]
  [T_1] -> DHW for ASHP Case/1(In1)
  Heat sys act?/1 -> Defrost Timer/2(In2)
  Delay1/1 -> Sum2/2
  Delay/1 -> Sum2/1
  [MassFlowTotal] -> Subsystem14/5(In5)
  Defrost Timer/2(Out2) -> [DefrostOn]
  DHW for ASHP Case/1(Out1) -> Scope2/1
  DHW for ASHP Case/7(Out7) -> [HeatToWater]
  DHW for ASHP Case/4(Out4) -> Sum3/2
  [DefrostOn] -> DHW for ASHP Case/4(In4)
  Subsystem14/3(Out3) -> Sum1/1
  DHW for ASHP Case/3(Out3) -> Sum1/2
  Sum3/1 -> Sum4/2, [n_signal]
  Defrost Timer/1(Out1) -> [NormalOn]
  Sum2/1 -> Saturation/1
  [DefrostOn] -> Subsystem14/3(In3)
  [T_Out] -> Defrost Timer/1(In1)
  [NormalOn] -> Subsystem14/2(In2)
  [NormalOn] -> DHW for ASHP Case/3(In3)
  DHW for ASHP Case/2(Out2) -> [DHW_heating_on]
  mains water temp/1 -> DHW for ASHP Case/6(In6)
  [DHW_heating_on] -> Logical Operator/1
  Logical Operator/1 -> [SH_Signal]

== system Final_EWASP_VC/ASHP_Subsystem_Variable ==
  DHW for ASHP Case : Subsystem
  Defrost Timer : Subsystem
  Delay : Delay  DelayLength=1  InitialCondition=0
  Delay1 : Delay  DelayLength=1  InitialCondition=0
  Delay2 : Delay  DelayLength=5  InitialCondition=0
  Discrete-Time Integrator : DiscreteIntegrator  ExternalReset=falling  SampleTime=-1  LimitOutput=on  UpperSaturationLimit=1  LowerSaturationLimit=0  ICPrevOutput=DiscIntNeverNeededParam  ICPrevScaledInput=DiscIntNeverNeededParam
  Divide : Product  Inputs=*/
  Heat sys act? : Constant
  Logical Operator : Logic  Operator=NOT  Inputs=1  AllPortsSameDT=off  OutDataTypeStr=boolean
  Saturation : Saturate  UpperLimit=1  LowerLimit=0
  Scope1 : Scope
  Scope16 : Scope  NumInputPorts=2
  Scope2 : Scope
  Scope3 : Scope
  Subsystem : Subsystem
      mask Display:
      | port_label('input', 1, 'T_outside')
      | port_label('input', 2, 'Normal_On')
      | port_label('input', 3, 'Defrost_On')
      | port_label('input', 4, 'returnTemp')
      | port_label('input', 5, 'm_dot_FullOn')
      | port_label('input', 6, 'GCS')
      | port_label('input', 7, 'SH')
      | 
      | port_label('output', 1, 'THB_to_Pre')
      | port_label('output', 2, 'Hysteresis')
      | port_label('output', 3, 'D_signal')
      | port_label('output', 4, 'N_signal')
      | port_label('output', 5, 'ElecOut')
      | port_label('output', 6, 'ThermOut')
  Sum1 : Sum
  Sum2 : Sum  Inputs=2
  Sum3 : Sum
  Sum4 : Sum
  Time in seconds for Heat pump to reach full stady state output : Constant  Value=pumpRamp
  Water Demand Time Series (Minute) : Constant  Value=DHWDemandProfile
  mains water temp : Constant  Value=12
  tag scope: AuxHeatToWater=global, DHW_heating_on=global, DefrostOn=global, ElectrifiedHeatToSpaceV=global, ElectrifiedHeatToWater=global, HeatToSpace=global, HeatToWater=global, NormalOn=global, SH_Signal=global, THB_In_Pre=global, d_signal=global, hysteresis=global, n_signal=global, pump_power_Fraction=global
  wires:
  [n_signal] -> Delay1/1
  Subsystem/2(Out2) -> [hysteresis]
  Sum1/1 -> Sum4/1, [d_signal]
  Saturation/1 -> Defrost Timer/3(In3)
  [d_signal] -> Delay/1
  [T_Out] -> Subsystem/1(In1)
  Subsystem/6(Out6) -> Scope16/1, [HeatToSpace]
  [SH_Signal] -> Subsystem/7(In7)
  DHW for ASHP Case/5(Out5) -> [ElectrifiedHeatToWater]
  [T_Out] -> DHW for ASHP Case/2(In2)
  DHW for ASHP Case/6(Out6) -> [AuxHeatToWater]
  Subsystem/1(Out1) -> Scope1/1, [THB_In_Pre]
  [MixedTemp] -> Subsystem/4(In4)
  Subsystem/4(Out4) -> Sum3/1
  Water Demand Time Series (Minute)/1 -> DHW for ASHP Case/5(In5)
  [Global_Control_Signal] -> Subsystem/6(In6)
  [T_1] -> DHW for ASHP Case/1(In1)
  Heat sys act?/1 -> Defrost Timer/2(In2)
  Delay1/1 -> Sum2/2
  Delay/1 -> Sum2/1
  [MassFlowTotal] -> Subsystem/5(In5)
  Defrost Timer/2(Out2) -> Scope3/1, [DefrostOn]
  DHW for ASHP Case/1(Out1) -> Scope2/1
  DHW for ASHP Case/7(Out7) -> [HeatToWater]
  DHW for ASHP Case/4(Out4) -> Sum3/2
  [DefrostOn] -> DHW for ASHP Case/4(In4)
  Subsystem/3(Out3) -> Sum1/1
  DHW for ASHP Case/3(Out3) -> Sum1/2
  Sum3/1 -> Sum4/2, [n_signal]
  Defrost Timer/1(Out1) -> [NormalOn]
  Sum2/1 -> Saturation/1
  [DefrostOn] -> Subsystem/3(In3)
  [T_Out] -> Defrost Timer/1(In1)
  [NormalOn] -> Subsystem/2(In2)
  [NormalOn] -> DHW for ASHP Case/3(In3)
  DHW for ASHP Case/2(Out2) -> [DHW_heating_on]
  mains water temp/1 -> DHW for ASHP Case/6(In6)
  [DHW_heating_on] -> Logical Operator/1
  Logical Operator/1 -> [SH_Signal]
  Discrete-Time Integrator/1 -> Delay2/1
  Sum4/1 -> Discrete-Time Integrator/2, Divide/1
  Delay2/1 -> [pump_power_Fraction]
  Time in seconds for Heat pump to reach full stady state output/1 -> Divide/2
  Divide/1 -> Discrete-Time Integrator/1
  [pump_power_Fraction] -> Subsystem/8(In8)
  Subsystem/5(Out5) -> Scope16/2, [ElectrifiedHeatToSpaceV]

== system Final_EWASP_VC/Airflow Model ==
  note: Select the correct state solution from
      | the 2 states that are simulated
  In1 : Inport
  In2 : Inport  Port=2
  In3 : Inport  Port=3
  In4 : Inport  Port=4
  In5 : Inport  Port=5
  Constant1 : Constant  Value=2
  Constant10 : Constant  Value=StateAirInEXPANDED_S
  Constant11 : Constant  Value=StateAirInEXPANDED_W
  Constant12 : Constant  Value=StateAirOutEXPANDED_S
  Constant13 : Constant  Value=StateAirOutEXPANDED_W
  Constant14 : Constant  Value=StateAirOutEXPANDED_N
  Constant15 : Constant  Value=StateAirOutEXPANDED_E
  Constant16 : Constant  Value=deltaPEXPANDED_N
  Constant17 : Constant  Value=deltaPEXPANDED_E
  Constant18 : Constant  Value=deltaPEXPANDED_S
  Constant19 : Constant  Value=deltaPEXPANDED_W
  Constant20 : Constant  Value=numRooms
  Constant21 : Constant  Value=buildingAge
  Constant23 : Constant  Value=StateAirInEXPANDED_S2
  Constant24 : Constant  Value=StateAirInEXPANDED_W2
  Constant25 : Constant  Value=StateAirOutEXPANDED_S2
  Constant26 : Constant  Value=StateAirOutEXPANDED_W2
  Constant27 : Constant  Value=StateAirOutEXPANDED_N2
  Constant28 : Constant  Value=StateAirOutEXPANDED_E2
  Constant29 : Constant  Value=deltaPEXPANDED_N2
  Constant3 : Constant  Value=buildingAge
  Constant30 : Constant  Value=deltaPEXPANDED_E2
  Constant31 : Constant  Value=deltaPEXPANDED_S2
  Constant32 : Constant  Value=deltaPEXPANDED_W2
  Constant33 : Constant  Value=[0;0;0;0;0;0;0;0;0;0;0]
  Constant34 : Constant  Value=numRooms
  Constant35 : Constant  Value=[0;0;0;0;0;0;0;0;0;0;0]
  Constant36 : Constant  Value=room2roomflowmatrix_N2
  Constant37 : Constant  Value=room2roomflowmatrix_E2
  Constant38 : Constant  Value=room2roomflowmatrix_S2
  Constant39 : Constant  Value=room2roomflowmatrix_W2
  Constant4 : Constant  Value=room2roomflowmatrix_N
  Constant40 : Constant  Value=StateAirInEXPANDED_N2
  Constant41 : Constant  Value=StateAirInEXPANDED_E2
  Constant42 : Constant  Value=[0;0;0;0;0;0;0;0;0;0;0]
  Constant5 : Constant  Value=room2roomflowmatrix_E
  Constant6 : Constant  Value=room2roomflowmatrix_S
  Constant7 : Constant  Value=room2roomflowmatrix_W
  Constant8 : Constant  Value=StateAirInEXPANDED_N
  Constant9 : Constant  Value=StateAirInEXPANDED_E
  Corrected buoyancy2 : Display  Commented=on
  Corrected buoyancy3 : Display  Commented=on
  MATLAB Function : MATLAB Function  TreatAsAtomicUnit=on
  MATLAB Function1 : MATLAB Function  TreatAsAtomicUnit=on
  Mean : dspstat3/Mean  run=off  InputProcessing=Columns as channels (frame based)  reset_popup=None  directionMode=Each column  dimension=1  roiEnable=off  roiType=Rectangles  roiPortion=Entire ROI  roiOutput=Individual statistics for each ROI  roiFlag=off  roundingMode=Floor  overflowMode=off  outputDataTypeStr=Inherit: Same as accumulator  outputMin=[]  outputMax=[]  outputLastDataTypeStr=Inherit: Same as accumulator
  Plus1 : Sum  Inputs=+-
  Plus3 : Sum
  Rate Transition{,1..5} (6 alike) : RateTransition  OutPortSampleTime=900
  Selector{1..2,4..5,7,13..16} (9 alike) : Selector  NumberOfDimensions=2  InputPortWidth=3  IndexOptions=Index vector (dialog),Index vector (dialog)  Indices=1:numRooms,1  OutputSizes=1,1
  Selector10 : Selector  NumberOfDimensions=2  InputPortWidth=3  IndexOptions=Index vector (dialog),Index vector (dialog)  Indices=1:11,1  OutputSizes=1,1
  Selector{3,6,11..12} (4 alike) : Selector  NumberOfDimensions=2  InputPortWidth=3  IndexOptions=Index vector (dialog),Index vector (dialog)  Indices=1:numRooms,1:numRooms  OutputSizes=1,1
  Selector8 : Selector  NumberOfDimensions=2  InputPortWidth=3  IndexOptions=Index vector (dialog),Index vector (dialog)  Indices=1:11,1  OutputSizes=1,1
  Selector9 : Selector  NumberOfDimensions=2  InputPortWidth=3  IndexOptions=Index vector (dialog),Index vector (dialog)  Indices=1:11,1  OutputSizes=1,1
  StateLoader : MATLAB Function  TreatAsAtomicUnit=on
  StateLoader1 : MATLAB Function  TreatAsAtomicUnit=on
  Subsystem1 : Subsystem  TreatAsAtomicUnit=on  SystemSampleTime=10
      mask Display:
      | port_label('input', 1, 'R2R_flow_matrix')
      | port_label('input', 2, 'Between_Floor_dP')
      | port_label('input', 3, 'Air_out_vector')
      | port_label('input', 4, 'Air_In_Vector')
      | port_label('input', 5, 'Room_Temp_Vector')
      | port_label('input', 6, 'Outdoor_Air_Temp')
      | 
      | port_label('output', 1, 'room_Convective_Heat_Gain')
  Subsystem2 : Subsystem  TreatAsAtomicUnit=on  SystemSampleTime=10
      mask Display:
      | port_label('input', 1, 'R2R_flow_matrix')
      | port_label('input', 2, 'Between_Floor_dP')
      | port_label('input', 3, 'Air_out_vector')
      | port_label('input', 4, 'Air_In_Vector')
      | port_label('input', 5, 'Room_Temp_Vector')
      | port_label('input', 6, 'Outdoor_Air_Temp')
      | 
      | port_label('output', 1, 'room_Convective_Heat_Gain')
  Switch : Switch  Threshold=2020  SaturateOnIntegerOverflow=off  InputSameDT=off
  Switch1 : Switch  Threshold=2020  SaturateOnIntegerOverflow=off  InputSameDT=off
  Switch2 : Switch  Criteria=u2 > Threshold  Threshold=1.5  SaturateOnIntegerOverflow=off  InputSameDT=off
  Vector Concatenate : Concatenate
  Vector Concatenate1 : Concatenate
  Out1 : Outport  VectorParamsAs1DForOutWhenUnconnected=off
  wires:
  [Wind_Speed] -> MATLAB Function/1(WindSpeed)
  Constant27/1 -> StateLoader1/12(StateAirOutEXPANDED_N)
  Selector1/1 -> [SAI_O]
  Constant15/1 -> StateLoader/13(StateAirOutEXPANDED_E)
  Constant19/1 -> StateLoader/19(deltaPEXPANDED_W)
  Constant9/1 -> StateLoader/9(StateAirInEXPANDED_E)
  Constant17/1 -> StateLoader/17(deltaPEXPANDED_E)
  Selector5/1 -> [SAO_O2]
  Constant26/1 -> StateLoader1/15(StateAirOutEXPANDED_W)
  Selector7/1 -> Corrected buoyancy3/1, Mean/1, [TVT]
  Subsystem1/1(Out1) -> Switch2/3
  Constant14/1 -> StateLoader/12(StateAirOutEXPANDED_N)
  Constant10/1 -> StateLoader/10(StateAirInEXPANDED_S)
  Subsystem2/1(Out1) -> Switch2/1
  [WindDir] -> MATLAB Function1/4(WindDir)
  [T_out] -> MATLAB Function1/3(T_out)
  StateLoader1/1(R2R_out) -> Selector11/1
  [Tin_Avg] -> MATLAB Function1/2(Tin_Avg)
  [R2R_Out] -> Subsystem1/1(In1)
  [Wind_Speed] -> MATLAB Function1/1(WindSpeed)
  Selector4/1 -> [SAI_O2]
  MATLAB Function1/3(DirIndex) -> StateLoader1/3(windDir)
  Constant31/1 -> StateLoader1/18(deltaPEXPANDED_S)
  Constant24/1 -> StateLoader1/11(StateAirInEXPANDED_W)
  MATLAB Function/2(StackIndex) -> Switch/3
  In4/1 -> [WindDir]
  Constant20/1 -> StateLoader/20(numRooms)
  Constant34/1 -> StateLoader1/20(numRooms)
  Constant5/1 -> StateLoader/5(room2roomflowmatrix_E)
  StateLoader1/2(StateAirIn_out) -> Selector13/1
  Constant6/1 -> StateLoader/6(room2roomflowmatrix_S)
  Constant38/1 -> StateLoader1/6(room2roomflowmatrix_S)
  [dP2] -> Subsystem2/2(In2)
  Constant29/1 -> StateLoader1/16(deltaPEXPANDED_N)
  Constant40/1 -> StateLoader1/8(StateAirInEXPANDED_N)
  Mean/1 -> [Tin_Avg], Corrected buoyancy2/1
  [WindDir] -> MATLAB Function/4(WindDir)
  Constant28/1 -> StateLoader1/13(StateAirOutEXPANDED_E)
  Constant32/1 -> StateLoader1/19(deltaPEXPANDED_W)
  Constant13/1 -> StateLoader/15(StateAirOutEXPANDED_W)
  [SAO_O] -> Subsystem1/3(In3)
  Constant36/1 -> StateLoader1/4(room2roomflowmatrix_N)
  Constant41/1 -> StateLoader1/9(StateAirInEXPANDED_E)
  [R2R_Out2] -> Subsystem2/1(In1)
  [SAO_O2] -> Subsystem2/3(In3)
  Constant23/1 -> StateLoader1/10(StateAirInEXPANDED_S)
  Constant30/1 -> StateLoader1/17(deltaPEXPANDED_E)
  Constant25/1 -> StateLoader1/14(StateAirOutEXPANDED_S)
  [SAI_O2] -> Subsystem2/4(In4)
  StateLoader1/4(deltaP) -> [dP2]
  Constant39/1 -> StateLoader1/7(room2roomflowmatrix_W)
  Constant8/1 -> StateLoader/8(StateAirInEXPANDED_N)
  Constant37/1 -> StateLoader1/5(room2roomflowmatrix_E)
  Selector6/1 -> [R2R_Out2]
  Constant12/1 -> StateLoader/14(StateAirOutEXPANDED_S)
  [dP] -> Subsystem1/2(In2)
  [T_out] -> Subsystem2/6(In6)
  MATLAB Function/1(WindIndex) -> StateLoader/1(windIndex)
  Constant7/1 -> StateLoader/7(room2roomflowmatrix_W)
  Constant16/1 -> StateLoader/16(deltaPEXPANDED_N)
  Selector2/1 -> [SAO_O]
  Constant4/1 -> StateLoader/4(room2roomflowmatrix_N)
  Constant11/1 -> StateLoader/11(StateAirInEXPANDED_W)
  [SAI_O] -> Subsystem1/4(In4)
  Selector3/1 -> [R2R_Out]
  Constant18/1 -> StateLoader/18(deltaPEXPANDED_S)
  MATLAB Function/3(DirIndex) -> StateLoader/3(windDir)
  [T_out] -> Subsystem1/6(In6)
  [Tin_Avg] -> MATLAB Function/2(Tin_Avg)
  [T_out] -> MATLAB Function/3(T_out)
  [TVT] -> Subsystem2/5(In5)
  In1/1 -> [Case_Switch]
  In2/1 -> [Wind_Speed]
  Switch2/1 -> Vector Concatenate/1
  In3/1 -> [T_out]
  In5/1 -> Selector7/1
  Constant35/1 -> Vector Concatenate/2
  Vector Concatenate/1 -> Selector8/1
  Selector8/1 -> Plus1/1
  Rate Transition/1 -> Selector2/1
  Rate Transition1/1 -> Selector3/1
  Rate Transition2/1 -> Selector1/1
  Rate Transition3/1 -> Selector6/1
  Rate Transition4/1 -> Selector4/1
  Rate Transition5/1 -> Selector5/1
  Plus3/1 -> Plus1/2
  Constant1/1 -> [mechIndex]
  [mechIndex] -> Switch/1
  Switch/1 -> StateLoader/2(stackIndex)
  Constant3/1 -> Switch/2
  MATLAB Function1/2(StackIndex) -> Switch1/3
  Switch1/1 -> StateLoader1/2(stackIndex)
  Constant21/1 -> Switch1/2
  [mechIndex] -> Switch1/1
  MATLAB Function1/1(WindIndex) -> StateLoader1/1(windIndex)
  [Case_Switch] -> Switch2/2
  [TVT] -> Vector Concatenate1/1
  Constant33/1 -> Vector Concatenate1/2
  Vector Concatenate1/1 -> Selector9/1
  Selector9/1 -> [TVTex]
  Constant42/1 -> Selector10/1
  Plus1/1 -> Out1/1
  Selector10/1 -> Plus3/2, Plus3/1
  [TVT] -> Subsystem1/5(In5)
  Selector11/1 -> Rate Transition3/1
  StateLoader/1(R2R_out) -> Selector12/1
  StateLoader/4(deltaP) -> [dP]
  Selector12/1 -> Rate Transition1/1
  Selector13/1 -> Rate Transition4/1
  StateLoader1/3(StateAirOut_out) -> Selector14/1
  Selector14/1 -> Rate Transition5/1
  Selector15/1 -> Rate Transition/1
  StateLoader/3(StateAirOut_out) -> Selector15/1
  StateLoader/2(StateAirIn_out) -> Selector16/1
  Selector16/1 -> Rate Transition2/1

== system Final_EWASP_VC/CondLossIntermediate ==
  In1 : Inport
  Constant3 : Constant
  Constant5 : Constant  Value=intermediateU*ceilingHeight*conductiveHconnectMatrix'
  Constant6 : Constant
  Direct Lookup Table (n-D) : LookupNDDirect  InputsSelectThisObjectFromTable=Vector  TableIsInput=on
  Direct Lookup Table (n-D)1 : LookupNDDirect  NumberOfTableDimensions=1  TableIsInput=on
  Mux : Mux  Inputs=11
  Product2 : Product
  Subtract : Sum  Inputs=+-
  Subtract1 : Sum  Inputs=+-
  Subtract2 : Sum  Inputs=+-
  Sum of Elements : Sum  Inputs=+
  per room loss : Display
  temp diff : Display
  Out1 : Outport  VectorParamsAs1DForOutWhenUnconnected=off
  wires:
  [T_4] -> Mux/4
  [T_9] -> Mux/9
  In1/1 -> Subtract1/1, Subtract2/1
  Constant6/1 -> Subtract2/2
  Constant5/1 -> Direct Lookup Table (n-D)/2
  Product2/1 -> Sum of Elements/1, per room loss/1
  Direct Lookup Table (n-D)/1 -> Product2/1
  [T_2] -> Mux/2
  [T_6] -> Mux/6
  [T_7] -> Mux/7
  Direct Lookup Table (n-D)1/1 -> Subtract/2
  [T_5] -> Mux/5
  [T_10] -> Mux/10
  Constant3/1 -> Subtract1/2
  [T_8] -> Mux/8
  Subtract2/1 -> Direct Lookup Table (n-D)1/1
  Mux/1 -> Direct Lookup Table (n-D)1/2, Subtract/1
  [T_11] -> Mux/11
  Subtract/1 -> Product2/2, temp diff/1
  [T_3] -> Mux/3
  [T_1] -> Mux/1
  Subtract1/1 -> Direct Lookup Table (n-D)/1
  Sum of Elements/1 -> Out1/1
